simulink model "kaskada_tran"  (R2015a)
settings: Solver=ode45  StartTime=0.0  StopTime=10.0  RelTol=1e-3
settings Model: Creator=Bojana Vasic  LastModifiedBy=Bojana Vasic

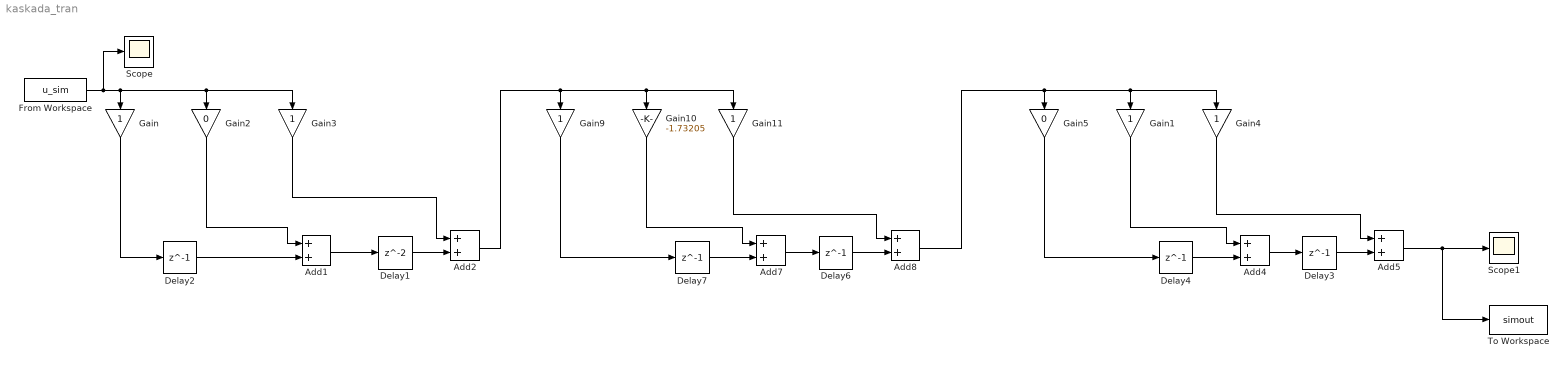
== system kaskada_tran ==
  Add{1..2,4..5,7..8} (6 alike) : Sum
  Delay1 : Delay
  Delay{2..4,6..7} (5 alike) : Delay  DelayLength=1
  From Workspace : FromWorkspace  VariableName=u_sim  SampleTime=1
  Gain{,1,3..4,9,11} (6 alike) : Gain
  Gain10 : Gain  Gain=-1.73205
  Gain2 : Gain  Gain=0
  Gain5 : Gain  Gain=0
  Scope : Scope
  Scope1 : Scope
  To Workspace : ToWorkspace  VariableName=simout  SaveFormat=Timeseries  SampleTime=-1
  wires:
  From Workspace/1 -> Scope/1, Gain3/1, Gain2/1, Gain/1
  Gain2/1 -> Add1/1
  Delay2/1 -> Add1/2
  Add1/1 -> Delay1/1
  Gain3/1 -> Add2/1
  Delay1/1 -> Add2/2
  Add2/1 -> Gain11/1, Gain10/1, Gain9/1
  Gain9/1 -> Delay7/1
  Gain10/1 -> Add7/1
  Delay7/1 -> Add7/2
  Add7/1 -> Delay6/1
  Gain11/1 -> Add8/1
  Delay6/1 -> Add8/2
  Add8/1 -> Gain4/1, Gain1/1, Gain5/1
  Gain1/1 -> Add4/1
  Delay4/1 -> Add4/2
  Add4/1 -> Delay3/1
  Gain4/1 -> Add5/1
  Delay3/1 -> Add5/2
  Gain/1 -> Delay2/1
  Gain5/1 -> Delay4/1
  Add5/1 -> To Workspace/1, Scope1/1
